simulink model "Scara"  (R2016b)
settings: Solver=VariableStepAuto  StartTime=0.0  StopTime=100  RelTol=1e-3
settings Model: Creator=Roozbeh  LastModifiedBy=Roozbeh

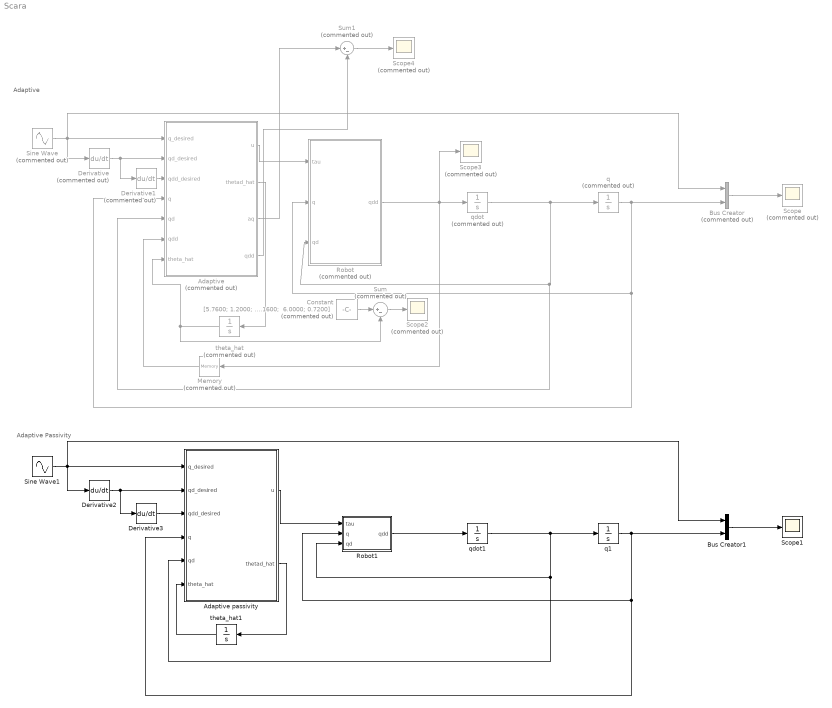
== system Scara ==
  note: Adaptive Passivity
  note: Adaptive
  Adaptive : MATLAB Function  Commented=on  TreatAsAtomicUnit=on
  Adaptive passivity : MATLAB Function  TreatAsAtomicUnit=on
  Bus Creator : BusCreator  Commented=on  Inputs=2
  Bus Creator1 : BusCreator  Inputs=2
  Constant : Constant  Commented=on  Value="[5.7600; 1.2000; 2.1600;  6.0000; 0.7200]"
  Derivative : Derivative  Commented=on
  Derivative1 : Derivative  Commented=on
  Derivative2 : Derivative
  Derivative3 : Derivative
  Memory : Memory  Commented=on  X0=zeros(3,1)
  Robot : MATLAB Function  Commented=on  TreatAsAtomicUnit=on
  Robot1 : MATLAB Function  TreatAsAtomicUnit=on
  Scope{,2..4} (4 alike) : Scope  Commented=on
  Scope1 : Scope
  Sine Wave : Sin  Commented=on  Amplitude=ones(3,1)*0  Bias=ones(3,1)*5  SampleTime=0
  Sine Wave1 : Sin  Amplitude=ones(3,1)*0  Bias=ones(3,1)*10  SampleTime=0
  Sum : Sum  Commented=on  Inputs=|+-
  Sum1 : Sum  Commented=on  Inputs=|+-
  q : Integrator  Commented=on  InitialCondition=[0 0 0]'
  q1 : Integrator  InitialCondition=[0 0 0]'
  qdot : Integrator  Commented=on  InitialCondition=[0 0 0]'
  qdot1 : Integrator  InitialCondition=[0 0 0]'
  theta_hat : Integrator  Commented=on  InitialCondition=|
      | [6.3038
      |     1.3461
      |     1.9183
      |     6.7441
      |     0.7486]'
  theta_hat1 : Integrator  InitialCondition=|
      | [5.6542
      |     1.1574
      |     2.3321
      |     6.5314
      |     0.6524]'
  wires:
  qdot/1 -> Adaptive/5(qd), Robot/3(qd), q/1
  q/1 -> Adaptive/4(q), Robot/2(q), Bus Creator/2
  theta_hat/1 -> Adaptive/7(theta_hat), Sum/2
  Sine Wave/1 -> Adaptive/1(q_desired), Bus Creator/1, Derivative/1
  Derivative/1 -> Adaptive/2(qd_desired), Derivative1/1
  Bus Creator/1 -> Scope/1
  Robot1/1(qdd) -> qdot1/1
  qdot1/1 -> q1/1, Robot1/3(qd), Adaptive passivity/5(qd)
  q1/1 -> Robot1/2(q), Adaptive passivity/4(q), Bus Creator1/2
  Adaptive passivity/1(u) -> Robot1/1(tau)
  Adaptive passivity/2(thetad_hat) -> theta_hat1/1
  theta_hat1/1 -> Adaptive passivity/6(theta_hat)
  Sine Wave1/1 -> Derivative2/1, Bus Creator1/1, Adaptive passivity/1(q_desired)
  Derivative2/1 -> Adaptive passivity/2(qd_desired), Derivative3/1
  Derivative3/1 -> Adaptive passivity/3(qdd_desired)
  Bus Creator1/1 -> Scope1/1
  Sum/1 -> Scope2/1
  Constant/1 -> Sum/1
  Adaptive/1(u) -> Robot/1(tau)
  Derivative1/1 -> Adaptive/3(qdd_desired)
  Adaptive/2(thetad_hat) -> theta_hat/1
  Robot/1(qdd) -> Memory/1, Scope3/1, qdot/1
  Memory/1 -> Adaptive/6("qdd ")
  Adaptive/3(aq) -> Sum1/1
  Adaptive/4(qdd) -> Sum1/2
  Sum1/1 -> Scope4/1

== matlab function Scara/Adaptive ==
  data: q_desired input; qd_desired input; qdd_desired input; q input; u output; qd input; qdd input; theta_hat input; thetad_hat output; aq output; qdd output
function [u, thetad_hat, aq, qdd] = fcn( q_desired, qd_desired, qdd_desired, q, qd, qdd, theta_hat)

g = 9.81;
q1 = q(1);
q2 = q(2);
q3 = q(3);

qd1 = qd(1);
qd2 = qd(2);
qd3 = qd(3);

e_q = q - q_desired;
e_qd = qd - qd_desired;

wn = 10;
Kd = eye(3)*wn^2;
Kp = eye(3)*2*wn;
aq = qdd_desired - Kd*e_qd - Kp*e_q;
qdd1 = aq(1);
qdd2 = aq(2);
qdd3 = aq(3);
Y = [qdd1 qdd1 + qdd2 2*qdd1*cos(q2) + qdd2*cos(q2) - 2*qd1*qd2*sin(q2) - 2*qd2^2*sin(q2) 0 qdd1 + qdd2; ...
    0 qdd1 + qdd2 qdd1*cos(q2) + qd1^2*sin(q2) 0 qdd1 + qdd2; 0 0 0 qdd3+g 0];


u = Y*theta_hat;

%update
e = [q; qd];
% A = [zeros(3) eye(3); -Kp -Kd];
B = [zeros(3); eye(3)];
% Q = eye(6);
% P = lyap(A,Q);
% wn = 1
%P = [1 0 0 -0.5 0 0; 0 1 0 0 -0.5 0; 0 0 1 0 0 -0.5; -0.5 0 0 1.5 0 0; 0 -0.5 0 0 1.5 0; 0 0 -0.5 0 0 1.5];
% wn = 10
P = [2.5053         0         0   -0.5000         0         0; ...
         0    2.5053         0         0   -0.5000         0; ...
         0         0    2.5053         0         0   -0.5000; ...
   -0.5000         0         0    0.1050         0         0; ...
         0   -0.5000         0         0    0.1050         0; ...
         0         0   -0.5000         0         0    0.1050]; 
% constructing Mhat
qdd1 = 1;
qdd2 = 0;
qdd3 = 0;
Mhat1 = [qdd1 qdd1 + qdd2 2*qdd1*cos(q2) + qdd2*cos(q2) 0 qdd1 + qdd2; ...
    0 qdd1 + qdd2 qdd1*cos(q2) 0 qdd1 + qdd2; 0 0 0 qdd3 0] * theta_hat;

qdd1 = 0;
qdd2 = 1;
qdd3 = 0;
Mhat2 = [qdd1 qdd1 + qdd2 2*qdd1*cos(q2) + qdd2*cos(q2) 0 qdd1 + qdd2; ...
    0 qdd1 + qdd2 qdd1*cos(q2) 0 qdd1 + qdd2; 0 0 0 qdd3 0] * theta_hat;

qdd1 = 0;
qdd2 = 0;
qdd3 = 1;
Mhat3 = [qdd1 qdd1 + qdd2 2*qdd1*cos(q2) + qdd2*cos(q2) 0 qdd1 + qdd2; ...
    0 qdd1 + qdd2 qdd1*cos(q2) 0 qdd1 + qdd2; 0 0 0 qdd3 0] * theta_hat;

Mhat = [transpose(Mhat1); transpose(Mhat2); transpose(Mhat3)];

qdd1 = qdd(1);
qdd2 = qdd(2);
qdd3 = qdd(3);
Yq = [qdd1 qdd1 + qdd2 2*qdd1*cos(q2) + qdd2*cos(q2) - 2*qd1*qd2*sin(q2) - 2*qd2^2*sin(q2) 0 qdd1 + qdd2; ...
    0 qdd1 + qdd2 qdd1*cos(q2) + qd1^2*sin(q2) 0 qdd1 + qdd2; 0 0 0 qdd3 0];


L = eye(5);
thetad_hat = -2*pinv(L)*transpose(pinv(Mhat)*Yq)*transpose(B)*P*e;

== matlab function Scara/Robot ==
  data: tau input; qdd output; q input; qd input
function qdd = fcn(tau, q, qd)

a1 = 0.6;
a2 = 0.4;

Lc1 = 0.3;
Lc2 = 0.2;

g = 9.81;
m1 = 12;
m2 = 6;
m3 = 6;
I1 = 0.36;
I2 = 0.36;
I3 = 0.36;

q1 = q(1);
q2 = q(2);
q3 = q(3);
qd1 = qd(1);
qd2 = qd(2);
qd3 = qd(3);

d11 = m1*Lc1^2 + m2*(a1^2 + Lc2^2 + 2*a1*Lc2*cos(q2)) + m3*(a1^2 + a2^2 + 2*a1*a2*cos(q2)) + I1 + I2 + I3;
d12 = m2*(Lc2^2 + a1*Lc2*cos(q2)) + m3*(a2^2 + a1*a2*cos(q2)) + I2 + I3;
d22 = m2*Lc2^2 + m3*a2^2 + I2 + I3;
d13 = 0;
d23 = 0;
d33 = m3;

D = [d11 d12 d13; d12 d22 d23; d13 d23 d33];

h = -m2*a1*Lc2*sin(q2) - m3*a1*a2*sin(q2);
C = [h*qd2 h*qd1+h*qd2 0; -h*qd1 0 0; 0 0 0];

G_mat = [0; 0; m3*g];

qdd = D\(tau - C*qd - G_mat);

== matlab function Scara/Adaptive passivity ==
  data: q_desired input; qd_desired input; qdd_desired input; q input; u output; qd input; theta_hat input; thetad_hat output
function [u, thetad_hat] = fcn( q_desired, qd_desired, qdd_desired, q, qd,theta_hat)

g = 9.81;
q1 = q(1);
q2 = q(2);
q3 = q(3);

qd1 = qd(1);
qd2 = qd(2);
qd3 = qd(3);

e_q = q - q_desired;
e_qd = qd - qd_desired;

gamma = eye(3);
v = qd_desired - gamma*e_q;
vd = qdd_desired - gamma*e_qd;
r = qd - v;

wn = 10;
Kd = eye(3)*wn^2;
Kp = eye(3)*2*wn;
qdd1 = vd(1);
qdd2 = vd(2);
qdd3 = vd(3);

Y = [qdd1 qdd1 + qdd2 2*qdd1*cos(q2) + qdd2*cos(q2) - v(1)*qd2*sin(q2) - qd1*v(2)*sin(q2) - 2*qd2*v(2)*sin(q2) 0 qdd1 + qdd2; ...
    0 qdd1 + qdd2 qdd1*cos(q2) + qd1*v(1)*sin(q2) 0 qdd1 + qdd2; 0 0 0 qdd3 + g 0];

K = 5*eye(3);
u = Y*theta_hat - K*r;

%update
L = eye(5)*0.2;
thetad_hat = -pinv(L)*transpose(Y)*r;

== matlab function Scara/Robot1 ==
  data: tau input; qdd output; q input; qd input
function qdd = fcn(tau, q, qd)

a1 = 0.6;
a2 = 0.4;

Lc1 = 0.3;
Lc2 = 0.2;

g = 9.81;
m1 = 12;
m2 = 6;
m3 = 6;
I1 = 0.36;
I2 = 0.36;
I3 = 0.36;

q1 = q(1);
q2 = q(2);
q3 = q(3);
qd1 = qd(1);
qd2 = qd(2);
qd3 = qd(3);

d11 = m1*Lc1^2 + m2*(a1^2 + Lc2^2 + 2*a1*Lc2*cos(q2)) + m3*(a1^2 + a2^2 + 2*a1*a2*cos(q2)) + I1 + I2 + I3;
d12 = m2*(Lc2^2 + a1*Lc2*cos(q2)) + m3*(a2^2 + a1*a2*cos(q2)) + I2 + I3;
d22 = m2*Lc2^2 + m3*a2^2 + I2 + I3;
d13 = 0;
d23 = 0;
d33 = m3;

D = [d11 d12 d13; d12 d22 d23; d13 d23 d33];

h = -m2*a1*Lc2*sin(q2) - m3*a1*a2*sin(q2);
C = [h*qd2 h*qd1+h*qd2 0; -h*qd1 0 0; 0 0 0];

G_mat = [0; 0; m3*g];

qdd = pinv(D)*(tau - C*qd - G_mat);
